simulink model "test_asbQuadcopter"  (R2021a)
settings: Solver=ode3  StartTime=0  StopTime=10  FixedStep=Ts  RelTol=1e-3  EnableMultiTasking=on
undefined symbols (not defined in the file or in its folder): Command, Desp_XYZ, FinalPos_XYZ, FinalPos_YPR, ft, init, InitPos_XYZ, InitPos_YPR, m, Noise_Amplitude, Noise_Chirp, Noise_Time, Pitch_Noise, Roll_Noise, s, steps_Pitch, steps_Roll, steps_X, steps_Y, steps_Yaw, steps_Z, takeOffDuration, Target_Time, time_stepsX, time_stepsY, time_stepsYaw, time_stepsZ, Time_Trans, Ts, Vehicle, Z_init, Z_Tesp
libraries: simulink x40, aerolibconvert2 x4, aerolibanimutils x2, SignalEditorBlockLib x2, environmentLibrary x2, sensorsLibrary x2, aerolibfltsims x2, aerolibutil x2, vrlib x1
(part 1 of 2)
settings Model: Creator=The MathWorks, Inc.  LastModifiedBy=Eduardo
settings SolverCC: AlgebraicLoopSolver=TrustRegion
settings DataIOCC: LimitDataPoints=on  SaveFormat=Array  SaveOutput=off  SignalLogging=off  DSMLogging=off  SaveTime=off
settings OptimizationCC: BlockReduction=off  BufferReuse=off  LifeSpan=inf
settings DebuggingCC: AlgebraicLoopMsg=none  ParameterPrecisionLossMsg=none  UnconnectedInputMsg=none  UnconnectedOutputMsg=none  UnconnectedLineMsg=none  AllowSymbolicDim=off  PregeneratedLibrarySubsystemCodeDiagnostic=none  SFUnexpectedBacktrackingDiag=warning  SFNoUnconditionalDefaultTransitionDiag=warning  SFExecutionAtInitializationDiag=none  SFMachineParentedDataDiag=warning  ArithmeticOperatorsInVariantConditions=warning
settings HardwareCC: ProdBitPerPointer=32  ProdBitPerSizeT=32  ProdBitPerPtrDiffT=32  ProdLargestAtomicFloat=None  ProdIntDivRoundTo=Undefined  ProdEndianess=Unspecified  ProdWordSize=32  ProdHWDeviceType=32-bit Generic
settings ModelReferenceCC: ModelReferenceNumInstancesAllowed=Single  PropagateSignalLabelsOutOfModel=off
settings SFSimCC: SimUseLocalCustomCode=off  CustomCodeUndefinedFunction=UseInterfaceOnly
settings RTWCC: RTWUseLocalCustomCode=off
settings CodeAppCC: StateflowObjectComments=on
settings GRTTargetCC: TargetLangStandard=C89/C90 (ANSI)
settings ConfigComp: CovMetricSettings=dw  CovSaveCumulativeToWorkspaceVar=on  CovSaveSingleToWorkspaceVar=on  CovExternalEMLEnable=off  CovSFcnEnable=off

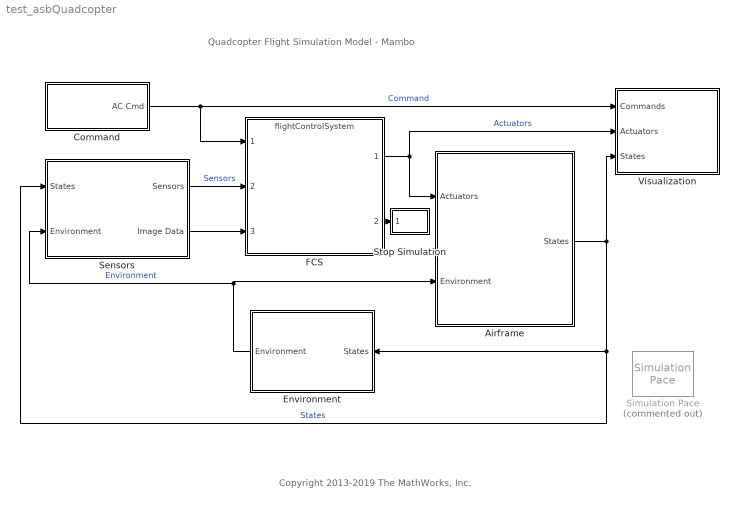
== system test_asbQuadcopter ==
  note: Quadcopter Flight Simulation Model - Mambo
  note: Copyright 2013-2019 The MathWorks, Inc.
  Airframe : Subsystem  Variant=on
  Command : Subsystem  Variant=on
  Environment : Subsystem  Variant=on
  FCS : ModelReference  ModelNameDialog=flightControlSystem.slx  SimulationMode=Normal  ModelReferenceVersion=2.2
  Sensors : Subsystem  Variant=on
  Simulation Pace : aerolibanimutils/Simulation Pace  Commented=on  SimulationPace=1  SleepMode=MATLAB Thread  OutputPaceError=off  SampleTime=Ts
      settings: AttributesFormatString=%<SimulationPace> sec/sec
  Stop Simulation : Subsystem
  Visualization : Subsystem
  wires:
  Command/1(AC Cmd) -> Visualization/1(Commands), FCS/1  "Command"
  Sensors/1(Sensors) -> FCS/2  "Sensors"
  FCS/1 -> Visualization/2(Actuators), Airframe/1(Actuators)  "Actuators"
  Environment/1(Environment) -> Airframe/2(Environment), Sensors/2(Environment)  "Environment"
  Airframe/1(States) -> Visualization/3(States), Environment/1(States), Sensors/1(States)  "States"
  FCS/2 -> Stop Simulation/1(Flags)
  Sensors/2(Image Data) -> FCS/3

== system test_asbQuadcopter/Airframe ==
  note: VSS_VEHICLE = 0 will select linear airframe
      | VSS_VEHICLE = 1 will select nonlnear airframe
  Actuators : Inport
  Environment : Inport  Port=2  OutDataTypeStr=Bus: EnvironmentBus
  Linear Airframe : ModelReference  ModelNameDialog=linearAirframe.slx  SimulationMode=Normal  VariantControl=VSS_VEHICLE_LINEAR  ModelReferenceVersion=1.41
  Nonlinear Airframe : ModelReference  ModelNameDialog=nonlinearAirframe.slx  SimulationMode=Normal  VariantControl=VSS_VEHICLE_NONLINEAR  ModelReferenceVersion=1.151
  States : Outport  OutDataTypeStr=Bus: StatesBus  VectorParamsAs1DForOutWhenUnconnected=off

== system test_asbQuadcopter/Command ==
  note: VSS_COMMAND = 0 will select Signal Editor
      | VSS_COMMAND = 1 will select Joystick + Signal Editor
      | VSS_COMMAND = 2 will select pre-saved data from .mat file
      | VSS_COMMAND = 3 will select pre-saved data from a spreadsheet
  Data : Subsystem  VariantControl=VSS_COMMAND_PRESAVED
  Joystick : Subsystem  VariantControl=VSS_COMMAND_JOYSTICK
  Signal Editor : Subsystem  VariantControl=VSS_COMMAND_SIGEDIT
  Spreadsheet Data : Subsystem  VariantControl=VSS_COMMAND_SPREADSHEET
  AC Cmd : Outport  OutDataTypeStr=Bus: CommandBus  VectorParamsAs1DForOutWhenUnconnected=off

== system test_asbQuadcopter/Environment ==
  note: VSS_ENVIRONMENT = 0 will select constant environment variables
      | VSS_ENVIRONMENT = 1 will select environment variables depending on position
  States : Inport  OutDataTypeStr=Bus: StatesBus
  Environment (Constant) : environmentLibrary/Environment (Constant)  SystemSampleTime=-1  VariantControl=VSS_ENVIRONMENT_CST  VariantActivationTime=update diagram  Latency=0  AutoFrameSizeCalculation=off
  Environment (Variable) : environmentLibrary/Environment (Variable)  SystemSampleTime=-1  VariantControl=VSS_ENVIRONMENT_VARIABLE  VariantActivationTime=update diagram  Latency=0  AutoFrameSizeCalculation=off
  Environment : Outport  OutDataTypeStr=Bus: EnvironmentBus  VectorParamsAs1DForOutWhenUnconnected=off

== system test_asbQuadcopter/Sensors ==
  note: VSS_SENSORS = 0 will select feedthrough sensors
      | VSS_SENSORS = 1 will select dynamics sensors with noise
  States : Inport
  Environment : Inport  Port=2
  Sensors (Dynamics) : sensorsLibrary/Sensors (Dynamics)  SystemSampleTime=-1  VariantControl=VSS_SENSORS_DYNAMICS  VariantActivationTime=update diagram  Latency=0  AutoFrameSizeCalculation=off
  Sensors (Feedthrough) : sensorsLibrary/Sensors (Feedthrough)  SystemSampleTime=-1  VariantControl=VSS_SENSORS_FEEDTHROUGH  VariantActivationTime=update diagram  Latency=0  AutoFrameSizeCalculation=off
  Sensors : Outport  VectorParamsAs1DForOutWhenUnconnected=off
  Image Data : Outport  Port=2  VectorParamsAs1DForOutWhenUnconnected=off

== system test_asbQuadcopter/Stop Simulation ==
  Flags : Inport  OutDataTypeStr=uint8
  Compare To Zero : simulink/Logic and Bit Operations/Compare To Zero  relop=>  OutDataTypeStr=boolean
  Flag has been triggered : Assertion
  Logical Operator : Logic  Operator=NOT  AllPortsSameDT=off  OutDataTypeStr=boolean
  wires:
  Flags/1 -> Compare To Zero/1
  Logical Operator/1 -> Flag has been triggered/1
  Compare To Zero/1 -> Logical Operator/1

== system test_asbQuadcopter/Visualization ==
  Commands : Inport
  Actuators : Inport  Port=2
  States : Inport  Port=3
  "Actuators " : InportShadow  Port=2
  Airspeed Indicator : AirspeedIndicatorBlock  LabelPosition=Hide  ScaleMin=0  ScaleMax=9
  Altimeter : AltimeterBlock  LabelPosition=Hide
  Artificial Horizon : ArtificialHorizonBlock  LabelPosition=Hide
  Climb Rate Indicator : ClimbIndicatorBlock  LabelPosition=Hide  ScaleMax=1000
  Extract Flight Instruments : Subsystem
  Heading Indicator : HeadingIndicatorBlock  LabelPosition=Hide
  "States " : InportShadow  Port=3
  Thruster {1..4} (4 alike) : RPMIndicatorBlock  LabelPosition=Hide
  Visualization : Subsystem  Commented=on  Variant=on
  wires:
  Actuators/1 -> Extract Flight Instruments/1(Actuators)
  States/1 -> Extract Flight Instruments/2(States)
  Commands/1 -> Visualization/2(Commands)
  "Actuators "/1 -> Visualization/3(Actuators)
  "States "/1 -> Visualization/1(States)

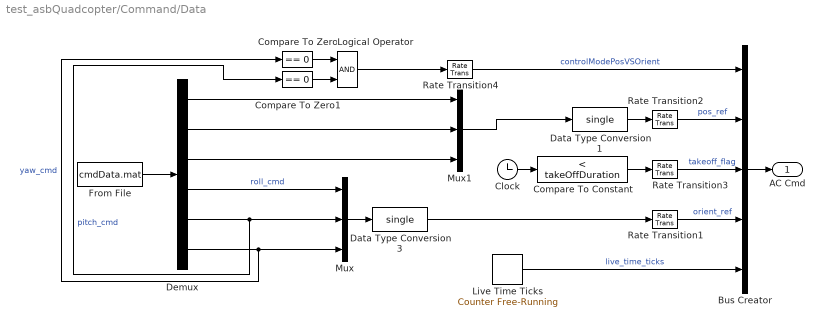
== system test_asbQuadcopter/Command/Data ==
  Bus Creator : BusCreator  Inputs=5  OutDataTypeStr=Bus: CommandBus  NonVirtualBus=on
  Clock : Clock
  Compare To Constant : simulink/Logic and Bit Operations/Compare To Constant  relop=<  const=takeOffDuration  OutDataTypeStr=boolean
  Compare To Zero : simulink/Logic and Bit Operations/Compare To Zero  relop===  OutDataTypeStr=boolean
  Compare To Zero1 : simulink/Logic and Bit Operations/Compare To Zero  relop===  OutDataTypeStr=boolean
  Data Type Conversion1 : DataTypeConversion  OutDataTypeStr=single
  Data Type Conversion3 : DataTypeConversion  OutDataTypeStr=single
  Demux : Demux  Outputs=6
  From File : FromFile  FileName=cmdData.mat  SampleTime=Ts
  Live Time Ticks : simulink/Sources/Counter Free-Running  NumBits=32  tsamp=Ts
  Logical Operator : Logic  IconShape=distinctive  AllPortsSameDT=off  OutDataTypeStr=boolean
  Mux : Mux  Inputs=3
  Mux1 : Mux  Inputs=3
  Rate Transition{1..4} (4 alike) : RateTransition  OutPortSampleTime=Ts
  AC Cmd : Outport  OutDataTypeStr=Bus: CommandBus  VectorParamsAs1DForOutWhenUnconnected=off
  wires:
  Demux/4 -> Mux/1  "roll_cmd"
  Demux/5 -> Mux/2, Compare To Zero1/1  "pitch_cmd"
  Demux/6 -> Compare To Zero/1, Mux/3  "yaw_cmd"
  From File/1 -> Demux/1
  Logical Operator/1 -> Rate Transition4/1
  Rate Transition1/1 -> Bus Creator/4  "orient_ref"
  Rate Transition2/1 -> Bus Creator/2  "pos_ref"
  Demux/3 -> Mux1/3
  Mux/1 -> Data Type Conversion3/1
  Data Type Conversion1/1 -> Rate Transition2/1
  Demux/1 -> Mux1/1
  Compare To Zero1/1 -> Logical Operator/2
  Compare To Zero/1 -> Logical Operator/1
  Mux1/1 -> Data Type Conversion1/1
  Clock/1 -> Compare To Constant/1
  Rate Transition4/1 -> Bus Creator/1  "controlModePosVSOrient"
  Data Type Conversion3/1 -> Rate Transition1/1
  Demux/2 -> Mux1/2
  Compare To Constant/1 -> Rate Transition3/1
  Rate Transition3/1 -> Bus Creator/3  "takeoff_flag"
  Live Time Ticks/1 -> Bus Creator/5  "live_time_ticks"
  Bus Creator/1 -> AC Cmd/1

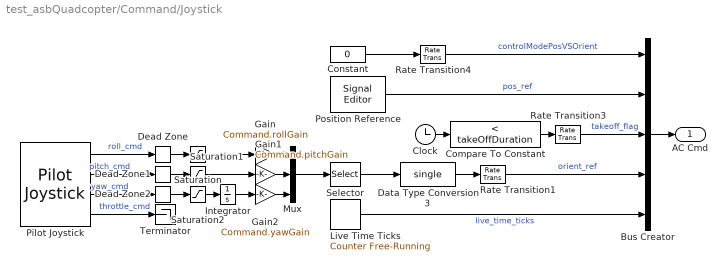
== system test_asbQuadcopter/Command/Joystick ==
  Bus Creator : BusCreator  Inputs=5  OutDataTypeStr=Bus: CommandBus  NonVirtualBus=on
  Clock : Clock
  Compare To Constant : simulink/Logic and Bit Operations/Compare To Constant  relop=<  const=takeOffDuration  OutDataTypeStr=boolean
  Constant : Constant  Value=0  OutDataTypeStr=boolean
  Data Type Conversion3 : DataTypeConversion  OutDataTypeStr=single
  Dead Zone : DeadZone  LowerValue=Command.rollDeadZoneStart  UpperValue=Command.rollDeadZoneEnd  SaturateOnIntegerOverflow=on
  Dead Zone1 : DeadZone  LowerValue=Command.pitchDeadZoneStart  UpperValue=Command.pitchDeadZoneEnd  SaturateOnIntegerOverflow=on
  Dead Zone2 : DeadZone  LowerValue=Command.yawDeadZoneStart  UpperValue=Command.yawDeadZoneEnd  SaturateOnIntegerOverflow=on
  Gain : Gain  Gain=Command.rollGain
  Gain1 : Gain  Gain=Command.pitchGain
  Gain2 : Gain  Gain=Command.yawGain
  Integrator : Integrator
  Live Time Ticks : simulink/Sources/Counter Free-Running  NumBits=32  tsamp=Ts
  Mux : Mux  Inputs=3
  Pilot Joystick : aerolibanimutils/Pilot Joystick  JoystickID=Joystick1  OutputConfiguration=FourAxis  SampleTime=Ts
  Position Reference : SignalEditorBlockLib/Signal Editor  FileName=positionRef.mat  ActiveScenario=Group1  ActiveSignal=XYZ  IsBus=off  OutputBusObjectStr=Bus: BusObject  SampleTime=Ts  Interpolate=off  ZeroCross=off  OutputAfterFinalValue=Setting to zero  Unit=inherit  PreserveSignalName=on
  Rate Transition1 : RateTransition  OutPortSampleTime=Ts
  Rate Transition3 : RateTransition  OutPortSampleTime=Ts
  Rate Transition4 : RateTransition  OutPortSampleTime=Ts
  Saturation : Saturate  UpperLimit=Command.rollSatUpper  LowerLimit=Command.rollSatLower
  Saturation1 : Saturate  UpperLimit=Command.pitchSatUpper  LowerLimit=Command.pitchSatLower
  Saturation2 : Saturate  UpperLimit=Command.yawSatUpper  LowerLimit=Command.yawSatLower
  Selector : Selector  InputPortWidth=3  IndexOptions=Index vector (dialog)  Indices=[3 2 1]  OutputSizes=1
  Terminator : Terminator
  AC Cmd : Outport  OutDataTypeStr=Bus: CommandBus  VectorParamsAs1DForOutWhenUnconnected=off
  wires:
  Pilot Joystick/4 -> Terminator/1  "throttle_cmd"
  Pilot Joystick/1 -> Dead Zone/1  "roll_cmd"
  Bus Creator/1 -> AC Cmd/1
  Constant/1 -> Rate Transition4/1
  Rate Transition1/1 -> Bus Creator/4  "orient_ref"
  Position Reference/1 -> Bus Creator/2  "pos_ref"
  Mux/1 -> Selector/1
  Compare To Constant/1 -> Rate Transition3/1
  Clock/1 -> Compare To Constant/1
  Rate Transition4/1 -> Bus Creator/1  "controlModePosVSOrient"
  Data Type Conversion3/1 -> Rate Transition1/1
  Pilot Joystick/2 -> Dead Zone1/1  "pitch_cmd"
  Rate Transition3/1 -> Bus Creator/3  "takeoff_flag"
  Live Time Ticks/1 -> Bus Creator/5  "live_time_ticks"
  Selector/1 -> Data Type Conversion3/1
  Dead Zone/1 -> Saturation/1
  Saturation/1 -> Gain/1
  Gain/1 -> Mux/1
  Dead Zone1/1 -> Saturation1/1
  Saturation1/1 -> Gain1/1
  Gain1/1 -> Mux/2
  Dead Zone2/1 -> Saturation2/1
  Saturation2/1 -> Integrator/1
  Gain2/1 -> Mux/3
  Pilot Joystick/3 -> Dead Zone2/1  "yaw_cmd"
  Integrator/1 -> Gain2/1

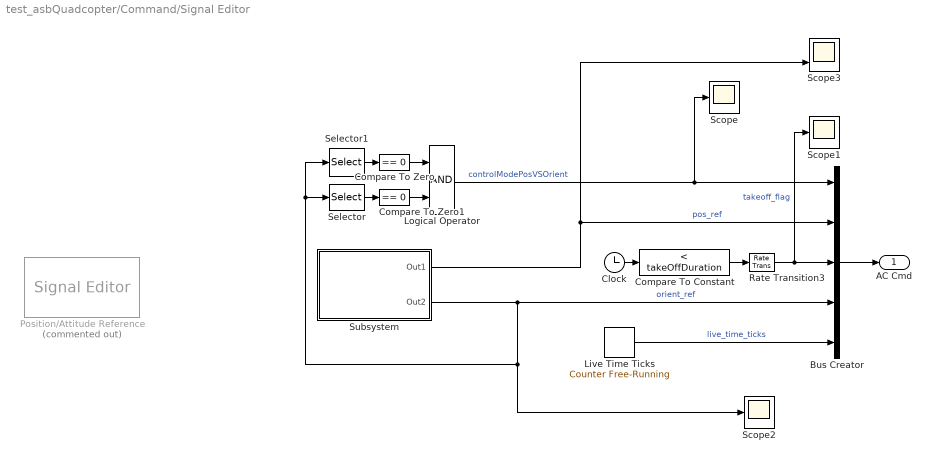
== system test_asbQuadcopter/Command/Signal Editor ==
  Bus Creator : BusCreator  Inputs=5  OutDataTypeStr=Bus: CommandBus  NonVirtualBus=on
  Clock : Clock
  Compare To Constant : simulink/Logic and Bit Operations/Compare To Constant  relop=<  const=takeOffDuration  OutDataTypeStr=boolean
  Compare To Zero : simulink/Logic and Bit Operations/Compare To Zero  relop===  OutDataTypeStr=boolean
  Compare To Zero1 : simulink/Logic and Bit Operations/Compare To Zero  relop===  OutDataTypeStr=boolean
  Live Time Ticks : simulink/Sources/Counter Free-Running  NumBits=32  tsamp=Ts
  Logical Operator : Logic  AllPortsSameDT=off  OutDataTypeStr=boolean
  Position/Attitude Reference : SignalEditorBlockLib/Signal Editor  Commented=on  FileName=positionAttitudeRef.mat  ActiveScenario=Hover  ActiveSignal=XYZ  IsBus=off  OutputBusObjectStr=Bus: BusObject  SampleTime=Ts  Interpolate=off  ZeroCross=off  OutputAfterFinalValue=Holding final value  Unit=inherit  PreserveSignalName=on
  Rate Transition3 : RateTransition  OutPortSampleTime=Ts
  Scope : Scope
  Scope1 : Scope
  Scope2 : Scope
  Scope3 : Scope  NumInputPorts=2
  Selector : Selector  InputPortWidth=3  IndexOptions=Index vector (dialog)  Indices=2  OutputSizes=1
  Selector1 : Selector  InputPortWidth=3  IndexOptions=Index vector (dialog)  Indices=3  OutputSizes=1
  Subsystem : Subsystem
  AC Cmd : Outport  OutDataTypeStr=Bus: CommandBus  VectorParamsAs1DForOutWhenUnconnected=off
  wires:
  Bus Creator/1 -> AC Cmd/1
  Compare To Zero/1 -> Logical Operator/1
  Compare To Zero1/1 -> Logical Operator/2
  Logical Operator/1 -> Scope/1, Bus Creator/1  "controlModePosVSOrient"
  Clock/1 -> Compare To Constant/1
  Compare To Constant/1 -> Rate Transition3/1
  Rate Transition3/1 -> Scope1/1, Bus Creator/3  "takeoff_flag"
  Live Time Ticks/1 -> Bus Creator/5  "live_time_ticks"
  Selector/1 -> Compare To Zero1/1
  Selector1/1 -> Compare To Zero/1
  Subsystem/2(Out2) -> Scope2/1, Selector1/1, Selector/1, Bus Creator/4  "orient_ref"
  Subsystem/1(Out1) -> Scope3/2, Bus Creator/2  "pos_ref"

== system test_asbQuadcopter/Command/Spreadsheet Data ==
  Bus Creator : BusCreator  Inputs=5  OutDataTypeStr=Bus: CommandBus  NonVirtualBus=on
  Clock : Clock
  Compare To Constant : simulink/Logic and Bit Operations/Compare To Constant  relop=<  const=takeOffDuration  OutDataTypeStr=boolean
  Compare To Zero : simulink/Logic and Bit Operations/Compare To Zero  relop===  OutDataTypeStr=boolean
  Compare To Zero1 : simulink/Logic and Bit Operations/Compare To Zero  relop===  OutDataTypeStr=boolean
  From Spreadsheet : FromSpreadsheet  FileName=cmdData.xlsx  SheetName=data  OutDataTypeStr=single  SampleTime=Ts
  Live Time Ticks : simulink/Sources/Counter Free-Running  NumBits=32  tsamp=Ts
  Logical Operator : Logic  IconShape=distinctive  AllPortsSameDT=off  OutDataTypeStr=boolean
  Mux : Mux  Inputs=3
  Mux1 : Mux  Inputs=3
  Rate Transition{1..4} (4 alike) : RateTransition  OutPortSampleTime=Ts
  AC Cmd : Outport  OutDataTypeStr=Bus: CommandBus  VectorParamsAs1DForOutWhenUnconnected=off
  wires:
  Bus Creator/1 -> AC Cmd/1
  From Spreadsheet/4 -> Mux/1  "roll_cmd"
  From Spreadsheet/6 -> Mux/3, Compare To Zero/1  "yaw_cmd"
  Logical Operator/1 -> Rate Transition4/1
  Rate Transition1/1 -> Bus Creator/4  "orient_ref"
  Rate Transition2/1 -> Bus Creator/2  "pos_ref"
  From Spreadsheet/3 -> Mux1/3
  Mux1/1 -> Rate Transition2/1
  From Spreadsheet/1 -> Mux1/1
  Compare To Zero1/1 -> Logical Operator/2
  Compare To Zero/1 -> Logical Operator/1
  Compare To Constant/1 -> Rate Transition3/1
  Clock/1 -> Compare To Constant/1
  Rate Transition4/1 -> Bus Creator/1  "controlModePosVSOrient"
  Mux/1 -> Rate Transition1/1
  From Spreadsheet/5 -> Mux/2, Compare To Zero1/1  "pitch_cmd"
  From Spreadsheet/2 -> Mux1/2
  Rate Transition3/1 -> Bus Creator/3  "takeoff_flag"
  Live Time Ticks/1 -> Bus Creator/5  "live_time_ticks"

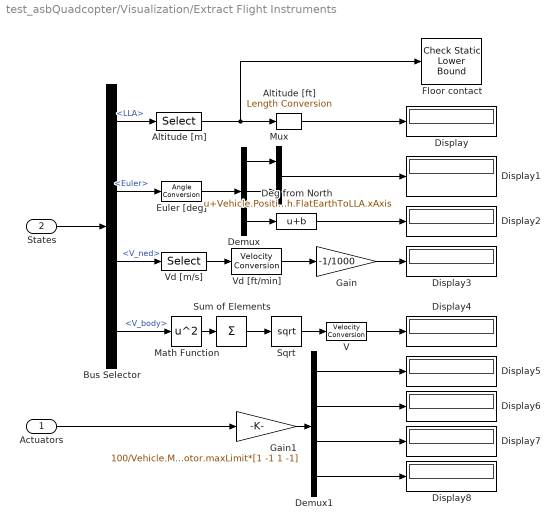
== system test_asbQuadcopter/Visualization/Extract Flight Instruments ==
  Actuators : Inport
  States : Inport  Port=2
  Altitude [ft] : aerolibconvert2/Length Conversion  IU=m  OU=ft
  Altitude [m] : Selector  InputPortWidth=3  IndexOptions=Index vector (dialog)  Indices=[3]  OutputSizes=1
  Bus Selector : BusSelector  OutputSignals=LLA,Euler,V_ned,V_body
  Deg from North : Bias  Bias=Vehicle.PositionOnEarth.FlatEarthToLLA.xAxis
  Demux : Demux  Outputs=3
  Demux1 : Demux
  Display{,1..8} (9 alike) : Display
  Euler [deg] : aerolibconvert2/Angle Conversion  IU=rad  OU=deg
  Floor contact : simulink/Model Verification/Check Static  Lower Bound  Description=init.posLLA(3) <= u  min=init.posLLA(3)  min_included=on  enabled=on  stopWhenAssertionFail=on  export=off  icon=graphic
  Gain : Gain  Gain=-1/1000
  Gain1 : Gain  Gain=100/Vehicle.Motor.maxLimit*[1 -1 1 -1]
  Math Function : Math  Operator=square  SignedPower=on  SaturateOnIntegerOverflow=on
  Mux : Mux  Inputs=2
  Sqrt : Sqrt  SaturateOnIntegerOverflow=on
  Sum of Elements : Sum  Inputs=+
  V : aerolibconvert2/Velocity Conversion  IU=m/s  OU=kts
  Vd [ft/min] : aerolibconvert2/Velocity Conversion  IU=m/s  OU=ft/min
  Vd [m/s] : Selector  InputPortWidth=3  IndexOptions=Index vector (dialog)  Indices=[3]  OutputSizes=1
  wires:
  Bus Selector/1 -> Altitude [m]/1  "<LLA>"
  Altitude [m]/1 -> Floor contact/1, Altitude [ft]/1
  States/1 -> Bus Selector/1
  Altitude [ft]/1 -> Display/1
  Bus Selector/2 -> Euler [deg]/1  "<Euler>"
  Euler [deg]/1 -> Demux/1
  Demux/1 -> Mux/1
  Demux/2 -> Mux/2
  Mux/1 -> Display1/1
  Deg from North/1 -> Display2/1
  Bus Selector/3 -> Vd [m/s]/1  "<V_ned>"
  Vd [m/s]/1 -> Vd [ft/min]/1
  Vd [ft/min]/1 -> Gain/1
  Gain/1 -> Display3/1
  Math Function/1 -> Sum of Elements/1
  Sum of Elements/1 -> Sqrt/1
  Bus Selector/4 -> Math Function/1  "<V_body>"
  Sqrt/1 -> V/1
  V/1 -> Display4/1
  Gain1/1 -> Demux1/1
  Demux1/1 -> Display5/1
  Demux1/2 -> Display6/1
  Demux1/3 -> Display7/1
  Demux1/4 -> Display8/1
  Actuators/1 -> Gain1/1
  Demux/3 -> Deg from North/1

== system test_asbQuadcopter/Visualization/Visualization ==
  note: VSS_VISUALIZATION = 0 will select scopes as means to visualie variables/states
      | VSS_VISUALIZATION = 1 will send select states in a variable to the workspace
      | VSS_VISUALIZATION = 2 will use FlightGear as visualization
      | VSS_VISUALIZATION = 3 will use a Simulink 3D interface
  States : Inport  OutDataTypeStr=Bus: StatesBus
  Commands : Inport  Port=2  OutDataTypeStr=Bus: CommandBus
  Actuators : Inport  Port=3
  FlightGear : Subsystem  VariantControl=VSS_VISUALIZATION_FLIGHTGEAR
      mask init:
      | visualizationFlightGearVars;
  Scopes : Subsystem  VariantControl=VSS_VISUALIZATION_SCOPES
  Simulink 3D : Subsystem  VariantControl=VSS_VISUALIZATION_SL3D
      mask init:
      | visualizationFlightGearVars;
  Workspace : Subsystem  VariantControl=VSS_VISUALIZATION_WORKSPACE

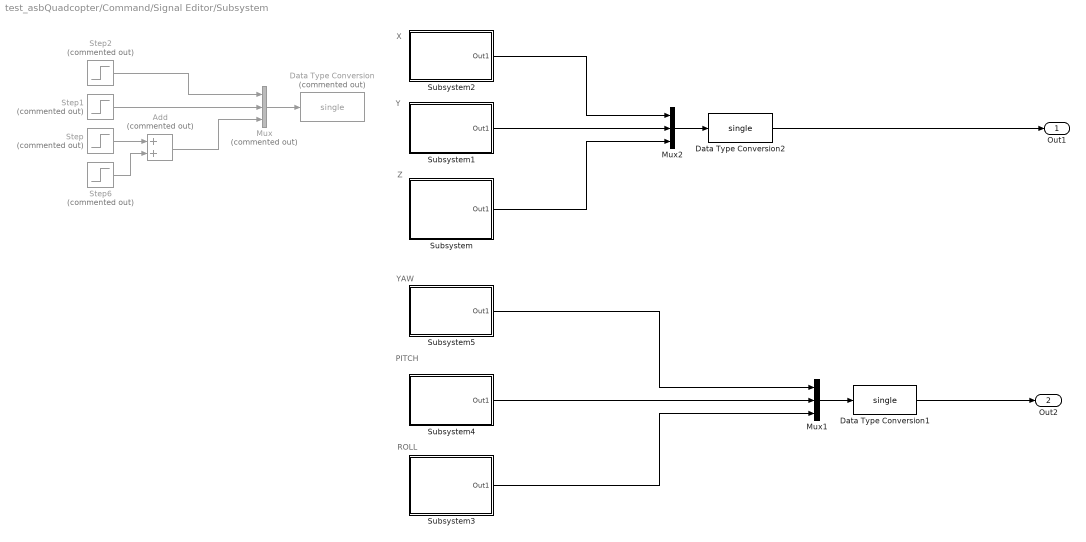
== system test_asbQuadcopter/Command/Signal Editor/Subsystem ==
  note: ROLL
  note: YAW
  note: PITCH
  note: Z
  note: X
  note: Y
  Add : Sum  Commented=on
  Data Type Conversion : DataTypeConversion  Commented=on  OutDataTypeStr=single
  Data Type Conversion1 : DataTypeConversion  OutDataTypeStr=single
  Data Type Conversion2 : DataTypeConversion  OutDataTypeStr=single
  Mux : Mux  Commented=on  Inputs=3
  Mux1 : Mux  Inputs=3
  Mux2 : Mux  Inputs=3
  Step : Step  Commented=on  Time=Time_Trans(2)  After=Desp_XYZ(3)  SampleTime=0
  Step1 : Step  Commented=on  Time=0  After=0  SampleTime=0
  Step2 : Step  Commented=on  Time=0  After=0  SampleTime=0
  Step6 : Step  Commented=on  After=-1.5  SampleTime=0
  Subsystem : Subsystem
  Subsystem1 : Subsystem
  Subsystem2 : Subsystem
  Subsystem3 : Subsystem
  Subsystem4 : Subsystem
  Subsystem5 : Subsystem
  Out1 : Outport
  Out2 : Outport  Port=2
  wires:
  Data Type Conversion2/1 -> Out1/1
  Data Type Conversion1/1 -> Out2/1
  Mux1/1 -> Data Type Conversion1/1
  Subsystem2/1(Out1) -> Mux2/1
  Mux2/1 -> Data Type Conversion2/1
  Subsystem/1(Out1) -> Mux2/3
  Subsystem1/1(Out1) -> Mux2/2
  Mux/1 -> Data Type Conversion/1
  Step/1 -> Add/1
  Add/1 -> Mux/3
  Step1/1 -> Mux/2
  Step2/1 -> Mux/1
  Step6/1 -> Add/2
  Subsystem5/1(Out1) -> Mux1/1
  Subsystem3/1(Out1) -> Mux1/3
  Subsystem4/1(Out1) -> Mux1/2

== system test_asbQuadcopter/Visualization/Visualization/FlightGear ==
  Commands : Inport
  States : Inport  Port=2
  Actuators : Inport  Port=3
  Bus Selector : BusSelector  OutputSignals=LLA,Euler
  FlightGear Preconfigured 6DoF Animation : aerolibfltsims/FlightGear Preconfigured 6DoF Animation  xFlightGearVersion=v2018.3  DestinationIpAddress=127.0.0.1  DestinationPort=Visualization.FlightGear.SixDOF.destinationPort  SampleTime=Ts  packetVersion=24
  Generate Run Script : aerolibfltsims/Generate Run Script  Architecture=Default  dataFlow=Send  GeometryModelName=Model  AirportId=KSFO  RunwayId=10L  InitialAltitude=Visualization.FlightGear.generateRunScript.initialAltitude  InitialHeading=Visualization.FlightGear.generateRunScript.initialHeading  OffsetDistance=Visualization.FlightGear.generateRunScript.offsetDistance  OffsetAzimuth=Visualization.FlightGear.generateRunScript.offsetAzimuth  InstallScenery=off  DisableShaders=off  OriginAddress=127.0.0.1  DestinationPort=Visualization.FlightGear.generateRunScript.destinationPort  OriginPort=5505  LocalAddress=127.0.0.1  OutputFileName=runfg.bat  FlightGearBaseDirectory=C:\Program Files\FlightGear
  Math Function : Math  Operator=transpose  SignedPower=on  SaturateOnIntegerOverflow=on
  Mux : Mux  Inputs=2
  Terminator : Terminator
  Terminator1 : Terminator
  wires:
  States/1 -> Bus Selector/1
  Bus Selector/2 -> Mux/2  "<Euler>"
  Mux/1 -> FlightGear Preconfigured 6DoF Animation/1
  Commands/1 -> Terminator/1
  Actuators/1 -> Terminator1/1
  Bus Selector/1 -> Math Function/1  "<LLA>"
  Math Function/1 -> Mux/1

== system test_asbQuadcopter/Visualization/Visualization/Scopes ==
  Commands : Inport
  States : Inport  Port=2
  Actuators : Inport  Port=3
  Bus Creator : BusCreator  Inputs=2
  Bus Selector : BusSelector  OutputSignals=States.V_body,States.Euler,States.X_ned
  Euler : Scope
  Terminator1 : Terminator
  V_body : Scope
  X_ned : Scope
  wires:
  Commands/1 -> Bus Creator/1  "Commands"
  States/1 -> Bus Creator/2  "States"
  Bus Creator/1 -> Bus Selector/1
  Bus Selector/1 -> V_body/1  "<V_body>"
  Bus Selector/2 -> Euler/1  "<Euler>"
  Bus Selector/3 -> X_ned/1  "<X_ned>"
  Actuators/1 -> Terminator1/1

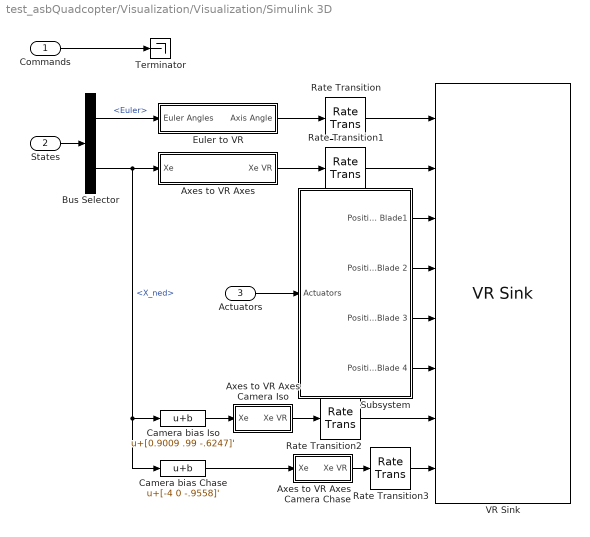
== system test_asbQuadcopter/Visualization/Visualization/Simulink 3D ==
  Commands : Inport
  States : Inport  Port=2
  Actuators : Inport  Port=3
  Axes to VR Axes : Subsystem
  Axes to VR Axes Camera Chase : Subsystem
  Axes to VR Axes Camera Iso : Subsystem
  Bus Selector : BusSelector  OutputSignals=Euler,X_ned
  Camera bias Chase : Bias  Bias=[-4 0 -.9558]'
  Camera bias Iso : Bias  Bias=[0.9009 .99 -.6247]'
  Euler to VR : Subsystem
  Rate Transition{,1..3} (4 alike) : RateTransition
  Subsystem : Subsystem
  Terminator : Terminator
  VR Sink : vrlib/VR Sink  InstantiateOnLoad=on  SampleTime=12*Ts  ViewEnable=on  RemoteChange=off  RemoteView=off  FieldsWritten=QuadBody.rotation.4.1.1.double#QuadBody.translation.3.1.1.double#Blade1.rotation.4.1.1.double#Blade3.rotation.4.1.1.double#Blade2.rotation.4.1.1.double#Blade4.rotation.4.1.1.double#IsoNoRotation.position.3.1.1.double#OnQuadNoRotation.position.3.1.1.double  WorldFileName=asbQuadcopterWorld.wrl  AutoView=on  VideoDimensions=[]  AllowVariableSize=off
  wires:
  Commands/1 -> Terminator/1
  Euler to VR/1(Axis Angle) -> Rate Transition/1
  Axes to VR Axes/1(Xe VR) -> Rate Transition1/1
  Bus Selector/1 -> Euler to VR/1(Euler Angles)  "<Euler>"
  Bus Selector/2 -> Camera bias Chase/1, Camera bias Iso/1, Axes to VR Axes/1(Xe)  "<X_ned>"
  States/1 -> Bus Selector/1
  Actuators/1 -> Subsystem/1(Actuators)
  Axes to VR Axes Camera Iso/1(Xe VR) -> Rate Transition2/1
  Camera bias Iso/1 -> Axes to VR Axes Camera Iso/1(Xe)
  Rate Transition/1 -> VR Sink/1
  Rate Transition1/1 -> VR Sink/2
  Subsystem/1(Position Blade1) -> VR Sink/3
  Subsystem/2(Position Blade 2) -> VR Sink/4
  Subsystem/3(Position Blade 3) -> VR Sink/5
  Subsystem/4(Position Blade 4) -> VR Sink/6
  Rate Transition2/1 -> VR Sink/7
  Axes to VR Axes Camera Chase/1(Xe VR) -> Rate Transition3/1
  Rate Transition3/1 -> VR Sink/8
  Camera bias Chase/1 -> Axes to VR Axes Camera Chase/1(Xe)

== system test_asbQuadcopter/Visualization/Visualization/Workspace ==
  Commands : Inport
  States : Inport  Port=2
  Actuators : Inport  Port=3
  Bus Selector : BusSelector  OutputSignals=V_body,Omega_body,Euler
  Bus Selector1 : BusSelector  OutputSignals=controlModePosVSOrient,pos_ref,takeoff_flag,orient_ref
  CommandsOut : ToWorkspace  VariableName=CommandsOut  SaveFormat=Structure With Time  SampleTime=-1
  Data Type Conversion{,1..3} (4 alike) : DataTypeConversion  OutDataTypeStr=double
  Mux : Mux  Inputs=3
  Mux1 : Mux
  StatesOut : ToWorkspace  VariableName=statesOut  SaveFormat=Structure With Time  SampleTime=-1
  Terminator1 : Terminator
  wires:
  States/1 -> Bus Selector/1
  Bus Selector/2 -> Mux/2  "<Omega_body>"
  Bus Selector/3 -> Mux/3  "<Euler>"
  Bus Selector/1 -> Mux/1  "<V_body>"
  Mux/1 -> StatesOut/1
  Commands/1 -> Bus Selector1/1
  Bus Selector1/2 -> Data Type Conversion1/1  "<pos_ref>"
  Bus Selector1/1 -> Data Type Conversion/1  "<controlModePosVSOrient>"
  Mux1/1 -> CommandsOut/1
  Bus Selector1/4 -> Data Type Conversion3/1  "<orient_ref>"
  Bus Selector1/3 -> Data Type Conversion2/1  "<takeoff_flag>"
  Actuators/1 -> Terminator1/1
  Data Type Conversion/1 -> Mux1/1
  Data Type Conversion1/1 -> Mux1/2
  Data Type Conversion2/1 -> Mux1/3
  Data Type Conversion3/1 -> Mux1/4

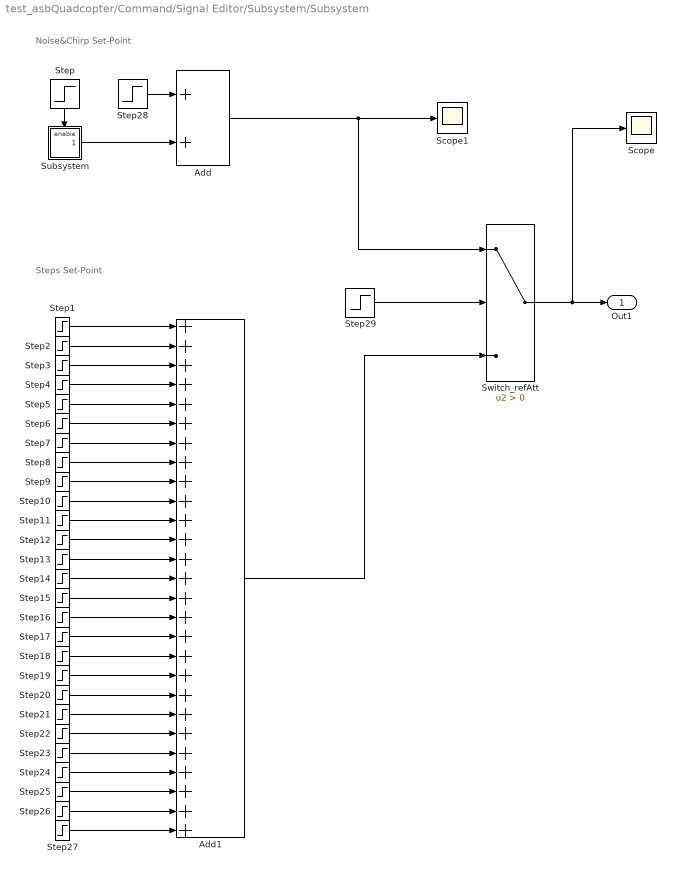
== system test_asbQuadcopter/Command/Signal Editor/Subsystem/Subsystem ==
  note: Noise&Chirp Set-Point
  note: Steps Set-Point
  Add : Sum
  Add1 : Sum  Inputs=+++++++++++++++++++++++++++
  Scope : Scope
  Scope1 : Scope
  Step : Step  Time=5  SampleTime=0
  Step1 : Step  After=Z_init  SampleTime=0
  Step10 : Step  Time=time_stepsZ(9)  After=steps_Z(9)  SampleTime=0
  Step11 : Step  Time=time_stepsZ(10)  After=steps_Z(10)  SampleTime=0
  Step12 : Step  Time=time_stepsZ(11)  After=steps_Z(11)  SampleTime=0
  Step13 : Step  Time=time_stepsZ(12)  After=steps_Z(12)  SampleTime=0
  Step14 : Step  Time=time_stepsZ(13)  After=steps_Z(13)  SampleTime=0
  Step15 : Step  Time=time_stepsZ(14)  After=steps_Z(14)  SampleTime=0
  Step16 : Step  Time=time_stepsZ(15)  After=steps_Z(15)  SampleTime=0
  Step17 : Step  Time=time_stepsZ(16)  After=steps_Z(16)  SampleTime=0
  Step18 : Step  Time=time_stepsZ(17)  After=steps_Z(17)  SampleTime=0
  Step19 : Step  Time=time_stepsZ(18)  After=steps_Z(18)  SampleTime=0
  Step2 : Step  Time=time_stepsZ(1)  After=steps_Z(1)  SampleTime=0
  Step20 : Step  Time=time_stepsZ(19)  After=steps_Z(19)  SampleTime=0
  Step21 : Step  Time=time_stepsZ(20)  After=steps_Z(20)  SampleTime=0
  Step22 : Step  Time=time_stepsZ(21)  After=steps_Z(21)  SampleTime=0
  Step23 : Step  Time=time_stepsZ(22)  After=steps_Z(22)  SampleTime=0
  Step24 : Step  Time=time_stepsZ(23)  After=steps_Z(23)
  Step25 : Step  Time=time_stepsZ(24)  After=steps_Z(24)
  Step26 : Step  Time=time_stepsZ(25)  After=steps_Z(25)
  Step27 : Step  Time=time_stepsZ(26)  After=steps_Z(26)
  Step28 : Step  After=Z_init  SampleTime=0
  Step29 : Step  Time=0  After=Z_Tesp  SampleTime=0
  Step3 : Step  Time=time_stepsZ(2)  After=steps_Z(2)  SampleTime=0
  Step4 : Step  Time=time_stepsZ(3)  After=steps_Z(3)  SampleTime=0
  Step5 : Step  Time=time_stepsZ(4)  After=steps_Z(4)  SampleTime=0
  Step6 : Step  Time=time_stepsZ(5)  After=steps_Z(5)  SampleTime=0
  Step7 : Step  Time=time_stepsZ(6)  After=steps_Z(6)  SampleTime=0
  Step8 : Step  Time=time_stepsZ(7)  After=steps_Z(7)  SampleTime=0
  Step9 : Step  Time=time_stepsZ(8)  After=steps_Z(8)  SampleTime=0
  Subsystem : Subsystem
  Switch_refAtt : Switch  Criteria=u2 > Threshold
  Out1 : Outport
  wires:
  Step14/1 -> Add1/14
  Step18/1 -> Add1/18
  Step16/1 -> Add1/16
  Step10/1 -> Add1/10
  Step11/1 -> Add1/11
  Step17/1 -> Add1/17
  Step20/1 -> Add1/20
  Step12/1 -> Add1/12
  Step13/1 -> Add1/13
  Step19/1 -> Add1/19
  Step15/1 -> Add1/15
  Step9/1 -> Add1/9
  Step2/1 -> Add1/2
  Step8/1 -> Add1/8
  Step21/1 -> Add1/21
  Step6/1 -> Add1/6
  Step4/1 -> Add1/4
  Step5/1 -> Add1/5
  Step3/1 -> Add1/3
  Step7/1 -> Add1/7
  Step1/1 -> Add1/1
  Add/1 -> Switch_refAtt/1, Scope1/1
  Step23/1 -> Add1/23
  Step22/1 -> Add1/22
  Step25/1 -> Add1/25
  Step24/1 -> Add1/24
  Step26/1 -> Add1/26
  Step27/1 -> Add1/27
  Add1/1 -> Switch_refAtt/3
  Switch_refAtt/1 -> Scope/1, Out1/1
  Step28/1 -> Add/1
  Subsystem/1(Out2) -> Add/2
  Step29/1 -> Switch_refAtt/2
  Step/1 -> Subsystem/Enable

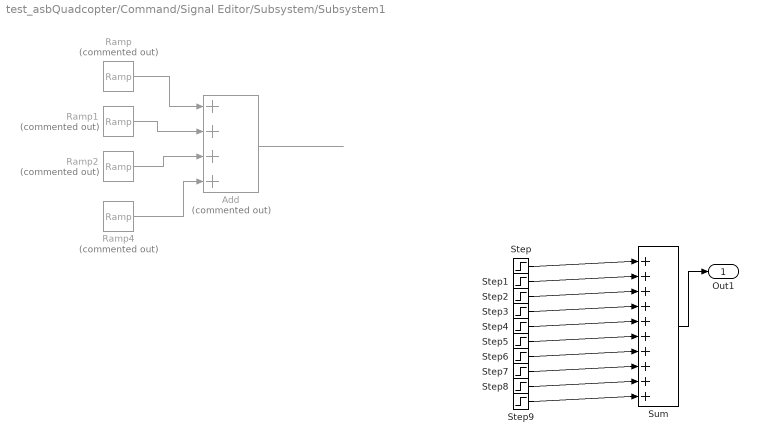
== system test_asbQuadcopter/Command/Signal Editor/Subsystem/Subsystem1 ==
  Add : Sum  Commented=on  Inputs=++++
  Ramp : simulink/Sources/Ramp  Commented=on  slope=InitPos_XYZ(2)/Time_Trans(1)  start=0  InitialOutput=0
  Ramp1 : simulink/Sources/Ramp  Commented=on  slope=-InitPos_XYZ(2)/Time_Trans(1)  start=Time_Trans(1)  InitialOutput=0
  Ramp2 : simulink/Sources/Ramp  Commented=on  slope=(InitPos_XYZ(2)-FinalPos_XYZ(2))/(Time_Trans(2)-Time_Trans(3))  start=Time_Trans(2)  InitialOutput=0
  Ramp4 : simulink/Sources/Ramp  Commented=on  slope=-(InitPos_XYZ(2)-FinalPos_XYZ(2))/(Time_Trans(2)-Time_Trans(3))  start=Time_Trans(3)  InitialOutput=0
  Step : Step  Time=time_stepsY(1)  After=steps_Y(1)  SampleTime=0
  Step1 : Step  Time=time_stepsY(2)  After=steps_Y(2)  SampleTime=0
  Step2 : Step  Time=time_stepsY(3)  After=steps_Y(3)  SampleTime=0
  Step3 : Step  Time=time_stepsY(4)  After=steps_Y(4)  SampleTime=0
  Step4 : Step  Time=time_stepsY(5)  After=steps_Y(5)  SampleTime=0
  Step5 : Step  Time=time_stepsY(6)  After=steps_Y(6)  SampleTime=0
  Step6 : Step  Time=time_stepsY(7)  After=steps_Y(7)  SampleTime=0
  Step7 : Step  Time=time_stepsY(8)  After=steps_Y(8)  SampleTime=0
  Step8 : Step  Time=time_stepsY(9)  After=steps_Y(9)  SampleTime=0
  Step9 : Step  Time=time_stepsY(10)  After=steps_Y(10)  SampleTime=0
  Sum : Sum  Inputs=|++++++++++
  Out1 : Outport
  wires:
  Add/1 -> ?
  Ramp4/1 -> Add/4
  Ramp1/1 -> Add/2
  Ramp/1 -> Add/1
  Ramp2/1 -> Add/3
  Sum/1 -> Out1/1
  Step/1 -> Sum/1
  Step1/1 -> Sum/2
  Step2/1 -> Sum/3
  Step3/1 -> Sum/4
  Step4/1 -> Sum/5
  Step5/1 -> Sum/6
  Step6/1 -> Sum/7
  Step7/1 -> Sum/8
  Step8/1 -> Sum/9
  Step9/1 -> Sum/10

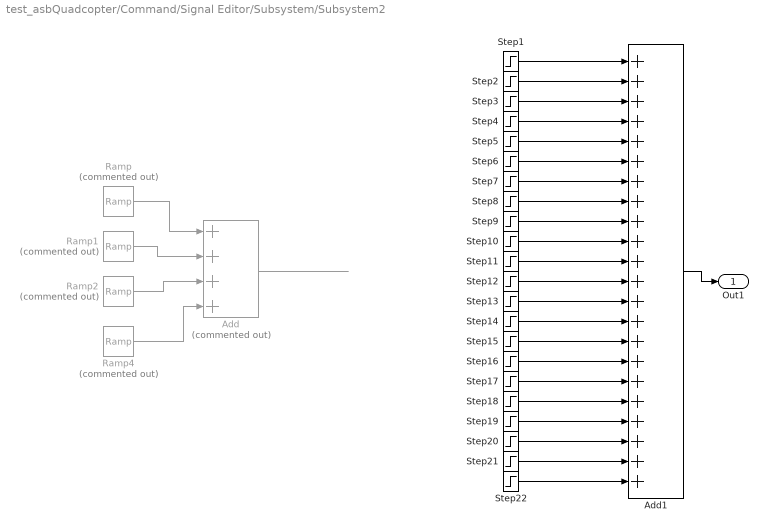
== system test_asbQuadcopter/Command/Signal Editor/Subsystem/Subsystem2 ==
  Add : Sum  Commented=on  Inputs=++++
  Add1 : Sum  Inputs=++++++++++++++++++++++
  Ramp : simulink/Sources/Ramp  Commented=on  slope=InitPos_XYZ(1)/Time_Trans(1)  start=0  InitialOutput=0
  Ramp1 : simulink/Sources/Ramp  Commented=on  slope=-InitPos_XYZ(1)/Time_Trans(1)  start=Time_Trans(1)  InitialOutput=0
  Ramp2 : simulink/Sources/Ramp  Commented=on  slope=(InitPos_XYZ(1)-FinalPos_XYZ(1))/(Time_Trans(2)-Time_Trans(3))  start=Time_Trans(2)  InitialOutput=0
  Ramp4 : simulink/Sources/Ramp  Commented=on  slope=-(InitPos_XYZ(1)-FinalPos_XYZ(1))/(Time_Trans(2)-Time_Trans(3))  start=Time_Trans(3)  InitialOutput=0
  Step1 : Step  Time=time_stepsX(1)  After=steps_X(1)  SampleTime=0
  Step10 : Step  Time=time_stepsX(10)  After=steps_X(10)  SampleTime=0
  Step11 : Step  Time=time_stepsX(11)  After=steps_X(11)  SampleTime=0
  Step12 : Step  Time=time_stepsX(12)  After=steps_X(12)  SampleTime=0
  Step13 : Step  Time=time_stepsX(13)  After=steps_X(13)  SampleTime=0
  Step14 : Step  Time=time_stepsX(14)  After=steps_X(14)  SampleTime=0
  Step15 : Step  Time=time_stepsX(15)  After=steps_X(15)  SampleTime=0
  Step16 : Step  Time=time_stepsX(16)  After=steps_X(16)  SampleTime=0
  Step17 : Step  Time=time_stepsX(17)  After=steps_X(17)  SampleTime=0
  Step18 : Step  Time=time_stepsX(18)  After=steps_X(18)  SampleTime=0
  Step19 : Step  Time=time_stepsX(19)  After=steps_X(19)  SampleTime=0
  Step2 : Step  Time=time_stepsX(2)  After=steps_X(2)  SampleTime=0
  Step20 : Step  Time=time_stepsX(20)  After=steps_X(20)  SampleTime=0
  Step21 : Step  Time=time_stepsX(21)  After=steps_X(21)  SampleTime=0
  Step22 : Step  Time=time_stepsX(22)  After=steps_X(22)  SampleTime=0
  Step3 : Step  Time=time_stepsX(3)  After=steps_X(3)  SampleTime=0
  Step4 : Step  Time=time_stepsX(4)  After=steps_X(4)  SampleTime=0
  Step5 : Step  Time=time_stepsX(5)  After=steps_X(5)  SampleTime=0
  Step6 : Step  Time=time_stepsX(6)  After=steps_X(6)  SampleTime=0
  Step7 : Step  Time=time_stepsX(7)  After=steps_X(7)  SampleTime=0
  Step8 : Step  Time=time_stepsX(8)  After=steps_X(8)  SampleTime=0
  Step9 : Step  Time=time_stepsX(9)  After=steps_X(9)  SampleTime=0
  Out1 : Outport
  wires:
  Add/1 -> ?
  Ramp1/1 -> Add/2
  Ramp4/1 -> Add/4
  Ramp/1 -> Add/1
  Ramp2/1 -> Add/3
  Step21/1 -> Add1/21
  Step7/1 -> Add1/7
  Step3/1 -> Add1/3
  Step6/1 -> Add1/6
  Add1/1 -> Out1/1
  Step4/1 -> Add1/4
  Step2/1 -> Add1/2
  Step15/1 -> Add1/15
  Step10/1 -> Add1/10
  Step13/1 -> Add1/13
  Step12/1 -> Add1/12
  Step8/1 -> Add1/8
  Step16/1 -> Add1/16
  Step17/1 -> Add1/17
  Step11/1 -> Add1/11
  Step22/1 -> Add1/22
  Step18/1 -> Add1/18
  Step14/1 -> Add1/14
  Step9/1 -> Add1/9
  Step20/1 -> Add1/20
  Step5/1 -> Add1/5
  Step1/1 -> Add1/1
  Step19/1 -> Add1/19

== system test_asbQuadcopter/Command/Signal Editor/Subsystem/Subsystem3 ==
  Add : Sum  Commented=on  Inputs=++++
  Add1 : Sum  Commented=on  Inputs=+++++++
  Ramp : simulink/Sources/Ramp  Commented=on  slope=InitPos_YPR(3)/Time_Trans(1)  start=0  InitialOutput=0
  Ramp1 : simulink/Sources/Ramp  Commented=on  slope=-InitPos_YPR(3)/Time_Trans(1)  start=Time_Trans(1)  InitialOutput=0
  Ramp2 : simulink/Sources/Ramp  Commented=on  slope=(InitPos_YPR(3)-FinalPos_YPR(3))/(Time_Trans(2)-Time_Trans(3))  start=Time_Trans(2)  InitialOutput=0
  Ramp4 : simulink/Sources/Ramp  Commented=on  slope=-(InitPos_YPR(3)-FinalPos_YPR(3))/(Time_Trans(2)-Time_Trans(3))  start=Time_Trans(3)  InitialOutput=0
  Step : Step  Commented=on  Time=5  After=0  SampleTime=0
  Step1 : Step  Commented=on  Time=20  After=steps_Roll(2)  SampleTime=0
  Step2 : Step  Commented=on  Time=35  After=steps_Roll(3)  SampleTime=0
  Step3 : Step  Commented=on  Time=50  After=steps_Roll(4)  SampleTime=0
  Step4 : Step  Commented=on  Time=65  After=steps_Roll(5)  SampleTime=0
  Step5 : Step  Commented=on  Time=80  After=steps_Roll(6)  SampleTime=0
  Step6 : Step  Commented=on  Time=95  After=steps_Roll(7)  SampleTime=0
  Step7 : Step  Commented=on  Time=5  After=Roll_Noise  SampleTime=0
  Subsystem : Subsystem  Commented=on
  Out1 : Outport
  wires:
  Ramp/1 -> Add/1
  Ramp1/1 -> Add/2
  Ramp2/1 -> Add/3
  Ramp4/1 -> Add/4
  Step1/1 -> Add1/2
  Add1/1 -> ?
  Step3/1 -> Add1/4
  Step4/1 -> Add1/5
  Step5/1 -> Add1/6
  Step2/1 -> Add1/3
  Step/1 -> Add1/1
  Step6/1 -> Add1/7
  Subsystem/1(Out1) -> Out1/1
  Step7/1 -> Subsystem/Enable

== system test_asbQuadcopter/Command/Signal Editor/Subsystem/Subsystem4 ==
  Add : Sum  Commented=on  Inputs=++++
  Add1 : Sum  Commented=on  Inputs=+++++++
  Ramp : simulink/Sources/Ramp  Commented=on  slope=InitPos_YPR(2)/Time_Trans(1)  start=0  InitialOutput=0
  Ramp1 : simulink/Sources/Ramp  Commented=on  slope=-InitPos_YPR(2)/Time_Trans(1)  start=Time_Trans(1)  InitialOutput=0
  Ramp2 : simulink/Sources/Ramp  Commented=on  slope=(InitPos_YPR(2)-FinalPos_YPR(2))/(Time_Trans(2)-Time_Trans(3))  start=Time_Trans(2)  InitialOutput=0
  Ramp4 : simulink/Sources/Ramp  Commented=on  slope=-(InitPos_YPR(2)-FinalPos_YPR(2))/(Time_Trans(2)-Time_Trans(3))  start=Time_Trans(3)  InitialOutput=0
  Step : Step  Commented=on  Time=5  After=0  SampleTime=0
  Step1 : Step  Commented=on  Time=20  After=steps_Pitch(2)  SampleTime=0
  Step2 : Step  Commented=on  Time=35  After=steps_Pitch(3)  SampleTime=0
  Step3 : Step  Commented=on  Time=50  After=steps_Pitch(4)  SampleTime=0
  Step4 : Step  Commented=on  Time=65  After=steps_Pitch(5)  SampleTime=0
  Step5 : Step  Commented=on  Time=80  After=steps_Pitch(6)  SampleTime=0
  Step6 : Step  Commented=on  Time=95  After=steps_Pitch(7)  SampleTime=0
  Step7 : Step  Commented=on  Time=5  After=Pitch_Noise  SampleTime=0
  Subsystem : Subsystem  Commented=on
  Out1 : Outport
  wires:
  Add/1 -> ?
  Ramp2/1 -> Add/3
  Ramp1/1 -> Add/2
  Ramp/1 -> Add/1
  Ramp4/1 -> Add/4
  Add1/1 -> ?
  Step/1 -> Add1/1
  Step1/1 -> Add1/2
  Step2/1 -> Add1/3
  Step3/1 -> Add1/4
  Step4/1 -> Add1/5
  Step5/1 -> Add1/6
  Step6/1 -> Add1/7
  Subsystem/1(Out1) -> Out1/1
  Step7/1 -> Subsystem/Enable

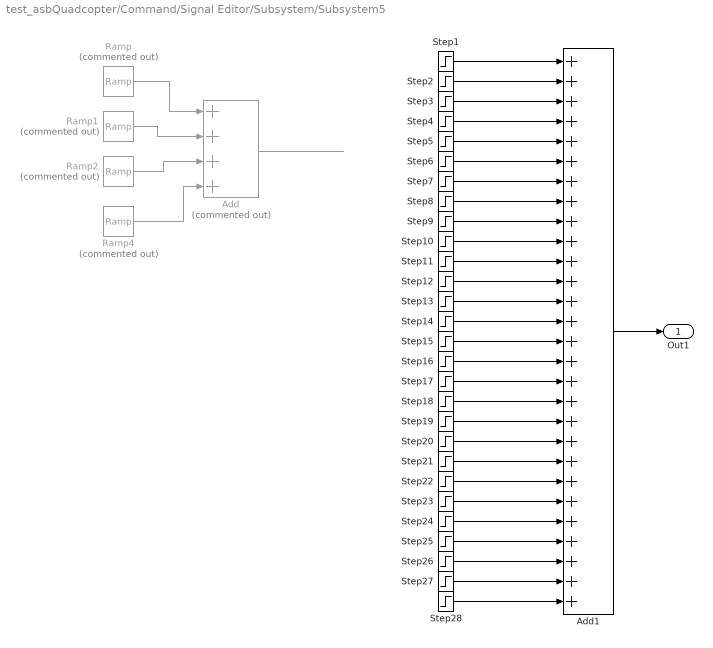
== system test_asbQuadcopter/Command/Signal Editor/Subsystem/Subsystem5 ==
  Add : Sum  Commented=on  Inputs=++++
  Add1 : Sum  Inputs=++++++++++++++++++++++++++++
  Ramp : simulink/Sources/Ramp  Commented=on  slope=InitPos_YPR(1)/Time_Trans(1)  start=0  InitialOutput=0
  Ramp1 : simulink/Sources/Ramp  Commented=on  slope=-InitPos_YPR(1)/Time_Trans(1)  start=Time_Trans(1)  InitialOutput=0
  Ramp2 : simulink/Sources/Ramp  Commented=on  slope=(InitPos_YPR(1)-FinalPos_YPR(1))/(Time_Trans(2)-Time_Trans(3))  start=Time_Trans(2)  InitialOutput=0
  Ramp4 : simulink/Sources/Ramp  Commented=on  slope=-(InitPos_YPR(1)-FinalPos_YPR(1))/(Time_Trans(2)-Time_Trans(3))  start=Time_Trans(3)  InitialOutput=0
  Step1 : Step  Time=time_stepsYaw(1)  After=steps_Yaw(1)  SampleTime=0
  Step10 : Step  Time=time_stepsYaw(10)  After=steps_Yaw(10)  SampleTime=0
  Step11 : Step  Time=time_stepsYaw(11)  After=steps_Yaw(11)  SampleTime=0
  Step12 : Step  Time=time_stepsYaw(12)  After=steps_Yaw(12)  SampleTime=0
  Step13 : Step  Time=time_stepsYaw(13)  After=steps_Yaw(13)  SampleTime=0
  Step14 : Step  Time=time_stepsYaw(14)  After=steps_Yaw(14)  SampleTime=0
  Step15 : Step  Time=time_stepsYaw(15)  After=steps_Yaw(15)  SampleTime=0
  Step16 : Step  Time=time_stepsYaw(16)  After=steps_Yaw(16)  SampleTime=0
  Step17 : Step  Time=time_stepsYaw(17)  After=steps_Yaw(17)  SampleTime=0
  Step18 : Step  Time=time_stepsYaw(18)  After=steps_Yaw(18)  SampleTime=0
  Step19 : Step  Time=time_stepsYaw(19)  After=steps_Yaw(19)  SampleTime=0
  Step2 : Step  Time=time_stepsYaw(2)  After=steps_Yaw(2)  SampleTime=0
  Step20 : Step  Time=time_stepsYaw(20)  After=steps_Yaw(20)  SampleTime=0
  Step21 : Step  Time=time_stepsYaw(21)  After=steps_Yaw(21)  SampleTime=0
  Step22 : Step  Time=time_stepsYaw(22)  After=steps_Yaw(22)  SampleTime=0
  Step23 : Step  Time=time_stepsYaw(23)  After=steps_Yaw(23)  SampleTime=0
  Step24 : Step  Time=time_stepsYaw(24)  After=steps_Yaw(24)  SampleTime=0
  Step25 : Step  Time=time_stepsYaw(25)  After=steps_Yaw(25)  SampleTime=0
  Step26 : Step  Time=time_stepsYaw(26)  After=steps_Yaw(26)  SampleTime=0
  Step27 : Step  Time=time_stepsYaw(27)  After=steps_Yaw(27)  SampleTime=0
  Step28 : Step  Time=time_stepsYaw(28)  After=steps_Yaw(28)  SampleTime=0
  Step3 : Step  Time=time_stepsYaw(3)  After=steps_Yaw(3)  SampleTime=0
  Step4 : Step  Time=time_stepsYaw(4)  After=steps_Yaw(4)  SampleTime=0
  Step5 : Step  Time=time_stepsYaw(5)  After=steps_Yaw(5)  SampleTime=0
  Step6 : Step  Time=time_stepsYaw(6)  After=steps_Yaw(6)  SampleTime=0
  Step7 : Step  Time=time_stepsYaw(7)  After=steps_Yaw(7)  SampleTime=0
  Step8 : Step  Time=time_stepsYaw(8)  After=steps_Yaw(8)  SampleTime=0
  Step9 : Step  Time=time_stepsYaw(9)  After=steps_Yaw(9)  SampleTime=0
  Out1 : Outport
  wires:
  Ramp1/1 -> Add/2
  Add/1 -> ?
  Ramp2/1 -> Add/3
  Ramp/1 -> Add/1
  Ramp4/1 -> Add/4
  Step5/1 -> Add1/5
  Step16/1 -> Add1/16
  Step20/1 -> Add1/20
  Step6/1 -> Add1/6
  Step18/1 -> Add1/18
  Step8/1 -> Add1/8
  Step19/1 -> Add1/19
  Step14/1 -> Add1/14
  Step13/1 -> Add1/13
  Step22/1 -> Add1/22
  Step1/1 -> Add1/1
  Step9/1 -> Add1/9
  Step11/1 -> Add1/11
  Step4/1 -> Add1/4
  Step10/1 -> Add1/10
  Step17/1 -> Add1/17
  Step15/1 -> Add1/15
  Step7/1 -> Add1/7
  Step3/1 -> Add1/3
  Step12/1 -> Add1/12
  Step21/1 -> Add1/21
  Step2/1 -> Add1/2
  Add1/1 -> Out1/1
  Step23/1 -> Add1/23
  Step24/1 -> Add1/24
  Step25/1 -> Add1/25
  Step26/1 -> Add1/26
  Step28/1 -> Add1/28
  Step27/1 -> Add1/27

== system test_asbQuadcopter/Visualization/Visualization/Simulink 3D/Axes to VR Axes ==
  Xe : Inport
  Demux : Demux  Outputs=3
      settings: DisplayOption=none
  Mux : Mux  Inputs=3
  rad-->deg1 : Gain  Gain=-1  SaturateOnIntegerOverflow=on  OutDataTypeStr=Inherit: Same as input  ParamDataTypeStr=Inherit: Same as input
  Xe VR : Outport  VectorParamsAs1DForOutWhenUnconnected=off
  wires:
  Xe/1 -> Demux/1
  Demux/1 -> Mux/1
  Demux/3 -> rad-->deg1/1
  Mux/1 -> Xe VR/1
  rad-->deg1/1 -> Mux/2
  Demux/2 -> Mux/3

== system test_asbQuadcopter/Visualization/Visualization/Simulink 3D/Axes to VR Axes Camera Chase ==
  Xe : Inport
  Demux : Demux  Outputs=3
      settings: DisplayOption=none
  Mux : Mux  Inputs=3
  rad-->deg1 : Gain  Gain=-1  SaturateOnIntegerOverflow=on  OutDataTypeStr=Inherit: Same as input  ParamDataTypeStr=Inherit: Same as input
  Xe VR : Outport  VectorParamsAs1DForOutWhenUnconnected=off
  wires:
  Xe/1 -> Demux/1
  Demux/1 -> Mux/1
  Demux/3 -> rad-->deg1/1
  Mux/1 -> Xe VR/1
  rad-->deg1/1 -> Mux/2
  Demux/2 -> Mux/3

== system test_asbQuadcopter/Visualization/Visualization/Simulink 3D/Axes to VR Axes Camera Iso ==
  Xe : Inport
  Demux : Demux  Outputs=3
      settings: DisplayOption=none
  Mux : Mux  Inputs=3
  rad-->deg1 : Gain  Gain=-1  SaturateOnIntegerOverflow=on  OutDataTypeStr=Inherit: Same as input  ParamDataTypeStr=Inherit: Same as input
  Xe VR : Outport  VectorParamsAs1DForOutWhenUnconnected=off
  wires:
  Demux/2 -> Mux/3
  rad-->deg1/1 -> Mux/2
  Mux/1 -> Xe VR/1
  Demux/3 -> rad-->deg1/1
  Demux/1 -> Mux/1
  Xe/1 -> Demux/1

== system test_asbQuadcopter/Visualization/Visualization/Simulink 3D/Euler to VR ==
  Euler Angles : Inport
  Axis Angle Vector : Subsystem
  Mux : Mux  Inputs=2
  Mux1 : Mux  Inputs=2
  Mux2 : Mux  Inputs=2
  Quaternion Multiplication (Pitch & Yaw) : aerolibutil/Quaternion Multiplication
  Quaternion Multiplication (Roll) : aerolibutil/Quaternion Multiplication
  Quaternion Normalization : Subsystem
  Quaternion Normalization1 : Subsystem
  Quaternion Normalization2 : Subsystem
  Selector : Selector  InputPortWidth=3  IndexOptions=Index vector (dialog)  Indices=[3]  OutputSizes=1
  Selector1 : Selector  InputPortWidth=3  IndexOptions=Index vector (dialog)  Indices=[2]  OutputSizes=1
  Selector2 : Selector  InputPortWidth=3  IndexOptions=Index vector (dialog)  Indices=[1]  OutputSizes=1
  Vr Pitch Axes : Constant  Value=[0 0 1]
  Vr Roll Axes : Constant  Value=[1 0 0]
  Vr Yaw Axes : Constant  Value=[0 -1 0]
  Axis Angle : Outport  VectorParamsAs1DForOutWhenUnconnected=off
  wires:
  Quaternion Multiplication (Roll)/1 -> Axis Angle Vector/1(e0)
  Axis Angle Vector/1(e0_norm) -> Axis Angle/1
  Quaternion Normalization/1(e0_norm) -> Quaternion Multiplication (Roll)/2
  Quaternion Normalization2/1(e0_norm) -> Quaternion Multiplication (Pitch & Yaw)/1
  Quaternion Normalization1/1(e0_norm) -> Quaternion Multiplication (Pitch & Yaw)/2
  Mux2/1 -> Quaternion Normalization2/1(e0)
  Mux1/1 -> Quaternion Normalization1/1(e0)
  Mux/1 -> Quaternion Normalization/1(e0)
  Selector/1 -> Mux2/1
  Vr Yaw Axes/1 -> Mux2/2
  Selector1/1 -> Mux1/1
  Vr Pitch Axes/1 -> Mux1/2
  Selector2/1 -> Mux/1
  Vr Roll Axes/1 -> Mux/2
  Euler Angles/1 -> Selector2/1, Selector1/1, Selector/1
  Quaternion Multiplication (Pitch & Yaw)/1 -> Quaternion Multiplication (Roll)/1

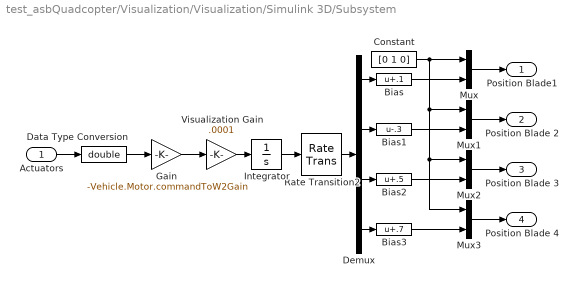
== system test_asbQuadcopter/Visualization/Visualization/Simulink 3D/Subsystem ==
  Actuators : Inport
  Bias : Bias  Bias=.1
  Bias1 : Bias  Bias=-.3
  Bias2 : Bias  Bias=.5
  Bias3 : Bias  Bias=.7
  Constant : Constant  Value=[0 1 0]
  Data Type Conversion : DataTypeConversion  OutDataTypeStr=double
  Demux : Demux
  Gain : Gain  Gain=-Vehicle.Motor.commandToW2Gain
  Integrator : Integrator  InitialCondition="[.1  .2 -.3 -.4]"  WrapState=on  WrappedStateUpperValue=2*pi  WrappedStateLowerValue=-2*pi
  Mux{,1..3} (4 alike) : Mux  Inputs=2
  Rate Transition2 : RateTransition
  Visualization Gain : Gain  Gain=.0001
  Position Blade1 : Outport  VectorParamsAs1DForOutWhenUnconnected=off
  Position Blade 2 : Outport  Port=2  VectorParamsAs1DForOutWhenUnconnected=off
  Position Blade 3 : Outport  Port=3  VectorParamsAs1DForOutWhenUnconnected=off
  Position Blade 4 : Outport  Port=4  VectorParamsAs1DForOutWhenUnconnected=off
  wires:
  Bias3/1 -> Mux3/2
  Mux3/1 -> Position Blade 4/1
  Bias1/1 -> Mux1/2
  Bias2/1 -> Mux2/2
  Demux/2 -> Bias1/1
  Visualization Gain/1 -> Integrator/1
  Constant/1 -> Mux3/1, Mux2/1, Mux1/1, Mux/1
  Mux1/1 -> Position Blade 2/1
  Mux2/1 -> Position Blade 3/1
  Data Type Conversion/1 -> Gain/1
  Integrator/1 -> Rate Transition2/1
  Mux/1 -> Position Blade1/1
  Gain/1 -> Visualization Gain/1
  Demux/3 -> Bias2/1
  Bias/1 -> Mux/2
  Actuators/1 -> Data Type Conversion/1
  Demux/4 -> Bias3/1
  Rate Transition2/1 -> Demux/1
  Demux/1 -> Bias/1

== system test_asbQuadcopter/Command/Signal Editor/Subsystem/Subsystem/Subsystem ==
  Enable : EnablePort
  Chirp Signal : simulink/Sources/Chirp Signal  f1=Initial_Freq  T=Target_Time  f2=Target_Freq
  ChirpFinish : Switch  Criteria=u2 > Threshold
  ChirpvsNoise : Switch  Criteria=u2 > Threshold
  Constant : Constant  Value=0
  Multiply : Gain  Gain=Noise_Amplitude
  Pulse Generator : DiscretePulseGenerator  PulseType=Time based  Period=Noise_Time  PulseWidth=40  PhaseDelay=10
  Scope1 : Scope
  Scope2 : Scope
  Step1 : Step  Time=Target_Time  Before=1  After=0  SampleTime=0
  Step29 : Step  Time=5  After=Noise_Chirp  SampleTime=0
  Subsystem : Subsystem
  Out2 : Outport
  wires:
  Step29/1 -> ChirpvsNoise/2
  ChirpvsNoise/1 -> Scope2/1, Out2/1
  Multiply/1 -> Scope1/1, ChirpvsNoise/1
  Chirp Signal/1 -> ChirpFinish/1
  ChirpFinish/1 -> ChirpvsNoise/3
  Constant/1 -> ChirpFinish/3
  Step1/1 -> ChirpFinish/2
  Subsystem/1(y) -> Multiply/1
  Pulse Generator/1 -> Subsystem/Enable

== system test_asbQuadcopter/Command/Signal Editor/Subsystem/Subsystem3/Subsystem ==
  Enable : EnablePort
  Multiply : Gain  Gain=Noise_Amplitude
  Pulse Generator : DiscretePulseGenerator  PulseType=Time based  Period=Noise_Time  PulseWidth=40  PhaseDelay=10
  Subsystem : Subsystem
  Out1 : Outport
  wires:
  Multiply/1 -> Out1/1
  Subsystem/1(y) -> Multiply/1
  Pulse Generator/1 -> Subsystem/Enable

== system test_asbQuadcopter/Command/Signal Editor/Subsystem/Subsystem4/Subsystem ==
  Enable : EnablePort
  Multiply : Gain  Gain=Noise_Amplitude
  Pulse Generator : DiscretePulseGenerator  PulseType=Time based  Period=Noise_Time  PulseWidth=40  PhaseDelay=10
  Subsystem : Subsystem
  Out1 : Outport
  wires:
  Multiply/1 -> Out1/1
  Subsystem/1(y) -> Multiply/1
  Pulse Generator/1 -> Subsystem/Enable

== system test_asbQuadcopter/Visualization/Visualization/Simulink 3D/Euler to VR/Axis Angle Vector ==
  e0 : Inport
  2 : Gain  Gain=2  SaturateOnIntegerOverflow=on  OutDataTypeStr=Inherit: Same as input  ParamDataTypeStr=Inherit: Same as input
  Constant : Constant  Value=1e-6
  Demux : Demux  Outputs=[1 3 ]
      settings: DisplayOption=none
  Mux : Mux  Inputs=2
  Product : Product  Inputs=*/  InputSameDT=on  SaturateOnIntegerOverflow=on  OutDataTypeStr=Inherit: Same as first input
  Switch : Switch  Criteria=u2 ~= 0
  Trigonometric Function : Trigonometry
  Trigonometric Function2 : Trigonometry  Operator=acos
  e0_norm : Outport  VectorParamsAs1DForOutWhenUnconnected=off
  wires:
  Demux/1 -> Trigonometric Function2/1
  Demux/2 -> Product/1
  Mux/1 -> e0_norm/1
  Product/1 -> Mux/1
  2/1 -> Mux/2
  Trigonometric Function/1 -> Switch/1, Switch/2
  Trigonometric Function2/1 -> Trigonometric Function/1, 2/1
  e0/1 -> Demux/1
  Constant/1 -> Switch/3
  Switch/1 -> Product/2

== system test_asbQuadcopter/Visualization/Visualization/Simulink 3D/Euler to VR/Quaternion Normalization ==
  e0 : Inport
  1/2 : Gain  Gain=1/2  SaturateOnIntegerOverflow=on  OutDataTypeStr=Inherit: Same as input  ParamDataTypeStr=Inherit: Same as input
  Demux : Demux  Outputs=[1 3]
      settings: DisplayOption=none
  Mux : Mux  Inputs=2
  Product : Product  InputSameDT=on  SaturateOnIntegerOverflow=on  OutDataTypeStr=Inherit: Same as first input
  Trigonometric Function : Trigonometry
  Trigonometric Function1 : Trigonometry  Operator=cos
  e0_norm : Outport  VectorParamsAs1DForOutWhenUnconnected=off
  wires:
  Trigonometric Function1/1 -> Mux/1
  Demux/2 -> Product/2
  Demux/1 -> 1/2/1
  Mux/1 -> e0_norm/1
  Product/1 -> Mux/2
  Trigonometric Function/1 -> Product/1
  1/2/1 -> Trigonometric Function1/1, Trigonometric Function/1
  e0/1 -> Demux/1

== system test_asbQuadcopter/Visualization/Visualization/Simulink 3D/Euler to VR/Quaternion Normalization1 ==
  e0 : Inport
  1/2 : Gain  Gain=1/2  SaturateOnIntegerOverflow=on  OutDataTypeStr=Inherit: Same as input  ParamDataTypeStr=Inherit: Same as input
  Demux : Demux  Outputs=[1 3]
      settings: DisplayOption=none
  Mux : Mux  Inputs=2
  Product : Product  InputSameDT=on  SaturateOnIntegerOverflow=on  OutDataTypeStr=Inherit: Same as first input
  Trigonometric Function : Trigonometry
  Trigonometric Function1 : Trigonometry  Operator=cos
  e0_norm : Outport  VectorParamsAs1DForOutWhenUnconnected=off
  wires:
  e0/1 -> Demux/1
  1/2/1 -> Trigonometric Function/1, Trigonometric Function1/1
  Trigonometric Function/1 -> Product/1
  Product/1 -> Mux/2
  Mux/1 -> e0_norm/1
  Demux/1 -> 1/2/1
  Demux/2 -> Product/2
  Trigonometric Function1/1 -> Mux/1
